simulink model "untitled"  (R2023a)
settings: Solver=VariableStepAuto  StartTime=0.0  StopTime=100.0  RelTol=1e-3
settings Model: Creator=BRL  LastModifiedBy=BRL

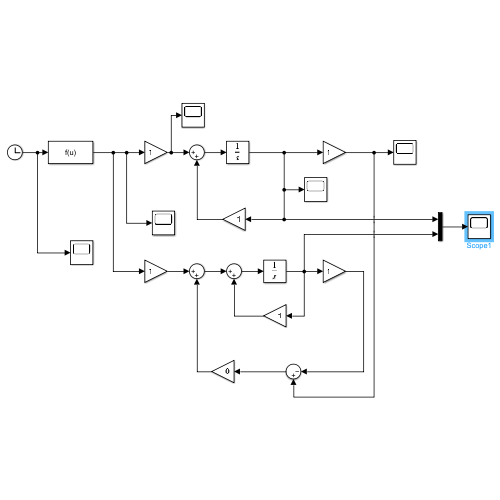
[thumbnail: Simulink's stored preview of the top-level diagram]
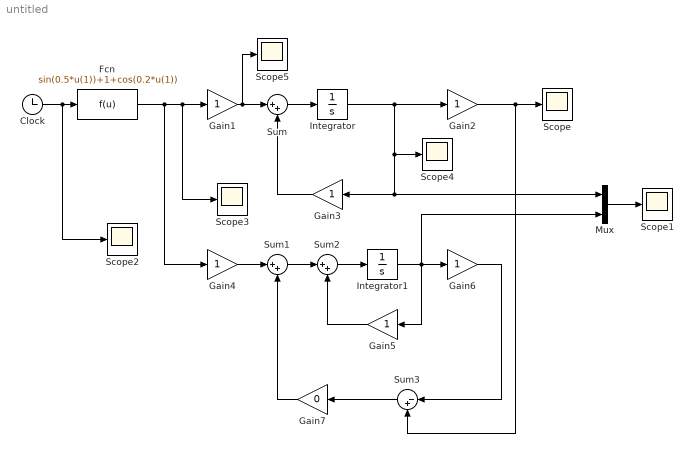
== system untitled ==
  Clock : Clock
  Fcn : Fcn  Expr=sin(0.5*u(1))+1+cos(0.2*u(1))
  Gain{1..6} (6 alike) : Gain
  Gain7 : Gain  Gain=0
  Integrator : Integrator
  Integrator1 : Integrator
  Mux : Mux  Inputs=2
  Scope{,1..5} (6 alike) : Scope
  Sum : Sum  Inputs=|++
  Sum1 : Sum  Inputs=|++
  Sum2 : Sum  Inputs=|++
  Sum3 : Sum  Inputs=|-+
  wires:
  Clock/1 -> Scope2/1, Fcn/1
  Fcn/1 -> Gain4/1, Scope3/1, Gain1/1
  Gain1/1 -> Scope5/1, Sum/1
  Sum/1 -> Integrator/1
  Integrator/1 -> Scope4/1, Mux/1, Gain3/1, Gain2/1
  Gain2/1 -> Sum3/2, Scope/1
  Gain3/1 -> Sum/2
  Gain4/1 -> Sum1/1
  Sum1/1 -> Sum2/1
  Sum2/1 -> Integrator1/1
  Gain5/1 -> Sum2/2
  Integrator1/1 -> Gain5/1, Mux/2, Gain6/1
  Mux/1 -> Scope1/1
  Gain6/1 -> Sum3/1
  Sum3/1 -> Gain7/1
  Gain7/1 -> Sum1/2
